simulink model "quadcopter1"  (R2014a)
settings: Solver=ode45  StartTime=0.0  StopTime=simTime  MaxStep=0.0001  RelTol=1e-3
settings Model: Creator=Ash  LastModifiedBy=Ash
settings DataIOCC: ExternalInput=Input  LimitDataPoints=off  LoadExternalInput=on  OutputSaveName=x_dd, y_dd, z_dd, gamma_d, beta_d, alpha_d, x, y, z, gamma, beta, alpha, x_d, y_d, z_d

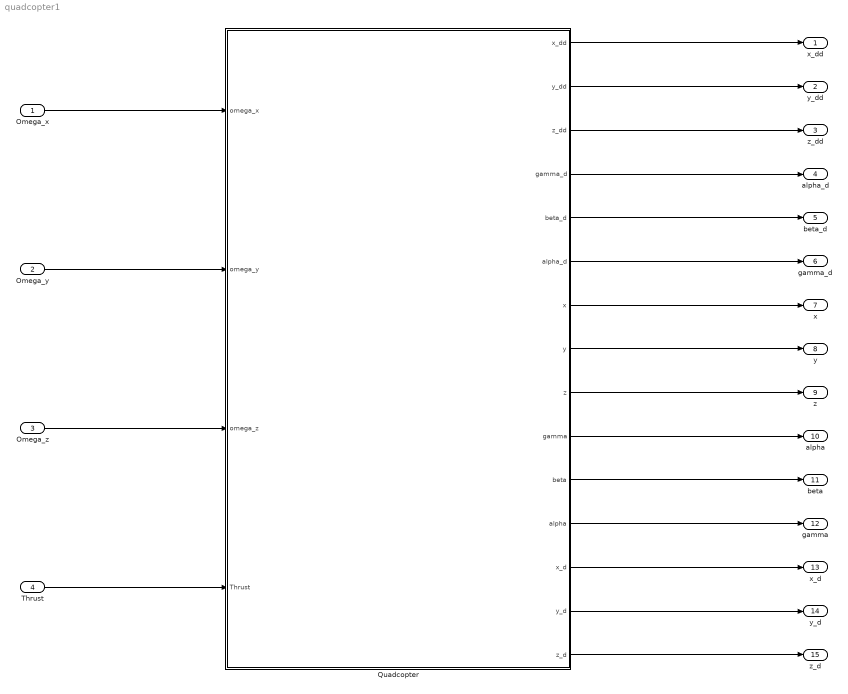
== system quadcopter1 ==
  Omega_x : Inport
  Omega_y : Inport  Port=2
  Omega_z : Inport  Port=3
  Thrust : Inport  Port=4
  Quadcopter : Subsystem
  x_dd : Outport
  y_dd : Outport  Port=2
  z_dd : Outport  Port=3
  alpha_d : Outport  Port=4
  beta_d : Outport  Port=5
  gamma_d : Outport  Port=6
  x : Outport  Port=7
  y : Outport  Port=8
  z : Outport  Port=9
  alpha : Outport  Port=10
  beta : Outport  Port=11
  gamma : Outport  Port=12
  x_d : Outport  Port=13
  y_d : Outport  Port=14
  z_d : Outport  Port=15
  wires:
  Quadcopter/1(x_dd) -> x_dd/1
  Quadcopter/2(y_dd) -> y_dd/1
  Omega_x/1 -> Quadcopter/1(omega_x)
  Omega_y/1 -> Quadcopter/2(omega_y)
  Omega_z/1 -> Quadcopter/3(omega_z)
  Thrust/1 -> Quadcopter/4(Thrust)
  Quadcopter/3(z_dd) -> z_dd/1
  Quadcopter/4(gamma_d) -> alpha_d/1
  Quadcopter/5(beta_d) -> beta_d/1
  Quadcopter/6(alpha_d) -> gamma_d/1
  Quadcopter/7(x) -> x/1
  Quadcopter/8(y) -> y/1
  Quadcopter/9(z) -> z/1
  Quadcopter/10(gamma) -> alpha/1
  Quadcopter/11(beta) -> beta/1
  Quadcopter/12(alpha) -> gamma/1
  Quadcopter/13(x_d) -> x_d/1
  Quadcopter/14(y_d) -> y_d/1
  Quadcopter/15(z_d) -> z_d/1

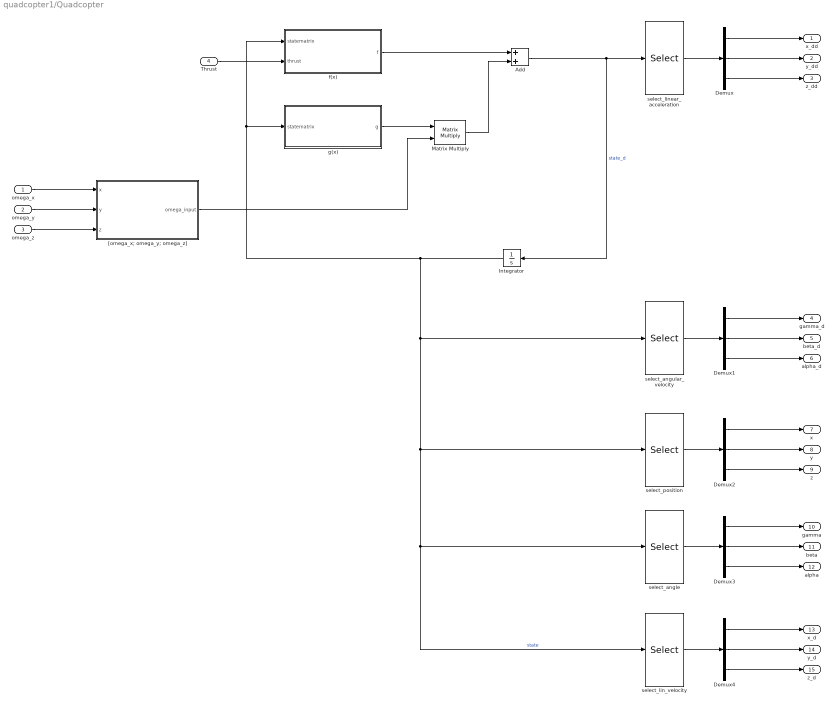
== system quadcopter1/Quadcopter ==
  omega_x : Inport
  omega_y : Inport  Port=2
  omega_z : Inport  Port=3
  Thrust : Inport  Port=4
  Add : Sum
  Demux{,1..4} (5 alike) : Demux  Outputs=[1 1 1]
  Integrator : Integrator
  Matrix Multiply : Product  Multiplication=Matrix(*)
  "[omega_x; omega_y; omega_z]" : MATLAB Function  TreatAsAtomicUnit=on
  f(x) : MATLAB Function  TreatAsAtomicUnit=on
  g(x) : MATLAB Function  TreatAsAtomicUnit=on
  select_angle : Selector  InputPortWidth=12  Indices=[7 9 11]
  select_angular_velocity : Selector  InputPortWidth=12  Indices=[8 10 12]
  select_lin_velocity : Selector  InputPortWidth=12  Indices=[2 4 6]
  select_linear_acceleration : Selector  InputPortWidth=12  Indices=[2 4 6]
  select_position : Selector  InputPortWidth=12  Indices=[1 3 5]
  x_dd : Outport
  y_dd : Outport  Port=2
  z_dd : Outport  Port=3
  gamma_d : Outport  Port=4
  beta_d : Outport  Port=5
  alpha_d : Outport  Port=6
  x : Outport  Port=7
  y : Outport  Port=8
  z : Outport  Port=9
  gamma : Outport  Port=10
  beta : Outport  Port=11
  alpha : Outport  Port=12
  x_d : Outport  Port=13
  y_d : Outport  Port=14
  z_d : Outport  Port=15
  wires:
  f(x)/1(f) -> Add/1
  Add/1 -> select_linear_acceleration/1, Integrator/1  "state_d"
  Matrix Multiply/1 -> Add/2
  "[omega_x; omega_y; omega_z]"/1(omega_input) -> Matrix Multiply/2
  g(x)/1(g) -> Matrix Multiply/1
  Thrust/1 -> f(x)/2(thrust)
  omega_z/1 -> "[omega_x; omega_y; omega_z]"/3(z)
  omega_y/1 -> "[omega_x; omega_y; omega_z]"/2(y)
  omega_x/1 -> "[omega_x; omega_y; omega_z]"/1(x)
  select_linear_acceleration/1 -> Demux/1
  Demux/1 -> x_dd/1
  Demux/2 -> y_dd/1
  Demux/3 -> z_dd/1
  select_angular_velocity/1 -> Demux1/1
  Demux1/1 -> gamma_d/1
  Demux1/2 -> beta_d/1
  Demux1/3 -> alpha_d/1
  select_position/1 -> Demux2/1
  Demux2/1 -> x/1
  Demux2/2 -> y/1
  Demux2/3 -> z/1
  select_angle/1 -> Demux3/1
  Demux3/1 -> gamma/1
  Demux3/2 -> beta/1
  Demux3/3 -> alpha/1
  Integrator/1 -> select_position/1, select_lin_velocity/1, select_angle/1, select_angular_velocity/1, f(x)/1(statematrix), g(x)/1(statematrix)  "state"
  select_lin_velocity/1 -> Demux4/1
  Demux4/1 -> x_d/1
  Demux4/2 -> y_d/1
  Demux4/3 -> z_d/1

== matlab function quadcopter1/Quadcopter/g(x) ==
  data: statematrix input; g output
function g = fcn(statematrix)

x = statematrix(1);
x_d = statematrix(2);
y = statematrix(3);
y_d = statematrix(4);
z = statematrix(5);
z_d = statematrix(6);
gamma = statematrix(7);
gamma_d = statematrix(8);
beta = statematrix(9);
beta_d = statematrix(10);
alpha = statematrix(11);
alpha_d = statematrix(12);

%new
g = [0 0 0; 0 0 0; 0 0 0; 0 0 0; 0 0 0; 0 0 0; 0 0 0; (cos(gamma)/(cos(beta)*cos(gamma)^2 + cos(beta)*sin(gamma)^2)) (sin(gamma)/(cos(beta)*cos(gamma)^2 + cos(beta)*sin(gamma)^2)) 0; 0 0 0; (-sin(gamma)/(cos(gamma)^2 + sin(gamma)^2)) (cos(gamma)/(cos(gamma)^2 + sin(gamma)^2)) 0; 0 0 0; ((cos(gamma)*sin(beta))/(cos(beta)*cos(gamma)^2 + cos(beta)*sin(gamma)^2)) ((sin(beta)*sin(gamma))/(cos(beta)*cos(gamma)^2 + cos(beta)*sin(gamma)^2)) 1];
%test
%g = [0 0 0; 0 0 0; 0 0 0; 0 0 0; 0 0 0; 0 0 0; 1 0 0; 1 0 0; 1 0 0; 1 0 0; 1 0 0; 1 0 0];

== matlab function quadcopter1/Quadcopter/f(x) ==
  data: statematrix input; f output; thrust input
function f = fcn(statematrix, thrust)

x = statematrix(1);
x_d = statematrix(2);
y = statematrix(3);
y_d = statematrix(4);
z = statematrix(5);
z_d = statematrix(6);
gamma = statematrix(7);
gamma_d = statematrix(8);
beta = statematrix(9);
beta_d = statematrix(10);
alpha = statematrix(11);
alpha_d = statematrix(12);

f = [x_d; thrust*(sin(alpha)*sin(gamma) + cos(alpha)*cos(gamma)*sin(beta)); y_d; -thrust*(cos(alpha)*sin(gamma) - cos(gamma)*sin(alpha)*sin(beta)); z_d; (thrust*cos(beta)*cos(gamma) - 9.81); gamma_d; 0; beta_d; 0; alpha_d; 0];

== matlab function quadcopter1/Quadcopter/[omega_x; omega_y; omega_z] ==
  data: x input; y input; z input; omega_input output
function omega_input = fcn(x, y ,z)

omega_input = [x; y; z];
